simulink model "quietdriver"  (R2024b)
settings: Solver=FixedStepAuto  StartTime=0.0  StopTime=100  RelTol=1e-3
libraries: robotlib x5
settings Model: Creator=sprinkle  LastModifiedBy=fafac
settings OptimizationCC: DefaultParameterBehavior=Inlined  EnhancedBackFolding=on  PassReuseOutputArgsAs=Individual arguments  ZeroExternalMemoryAtStartup=off  ZeroInternalMemoryAtStartup=off  MaxStackSize=64  OptimizeBlockOrder=speed  DifferentSizesBufferReuse=on  OptimizationCustomize=off  EfficientTunableParamExpr=on
settings DebuggingCC: ParameterTunabilityLossMsg=error
settings HardwareCC: ProdBitPerPointer=32  ProdBitPerSizeT=32  ProdBitPerPtrDiffT=32  ProdLargestAtomicFloat=None  ProdIntDivRoundTo=Undefined  ProdEndianess=Unspecified  ProdWordSize=32  ProdHWDeviceType=Generic->Unspecified (assume 32-bit Generic)
settings SFSimCC: MATLABDynamicMemAlloc=off  SimTargetLang=C++
settings RTWCC: Description=Embedded Coder  SystemTargetFile=ert.tlc  HardwareBoard=Robot Operating System (ROS)  TLCOptions="-aInlineSetEventsForThisBaseRateFcn=TLC_FALSE -aSuppressMultiTaskScheduler=TLC_FALSE  -aRateBasedStepFcn=0"  TemplateMakefile=ert_default_tmf  Toolchain=Catkin  TargetLang=C++  GPUComputeCapability=3.5
settings CodeAppCC: ForceParamTrailComments=on  IgnoreCustomStorageClasses=off  OperatorAnnotations=on  SimulinkDataObjDesc=on  SFDataObjDesc=on  InsertBlockDesc=on
settings ERTTargetCC: CodeInterfacePackaging=C++ class  SupportContinuousTime=on  RootIOFormat=Structure reference

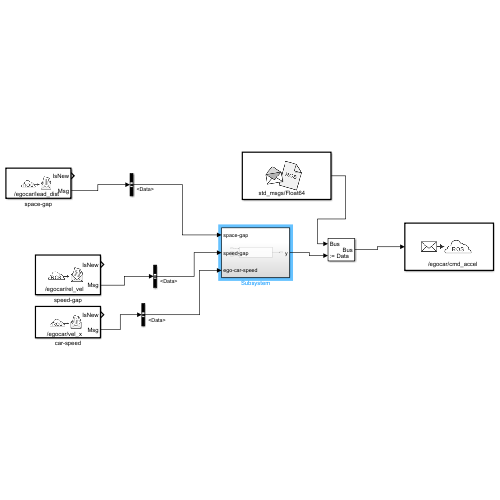
[thumbnail: Simulink's stored preview of the top-level diagram]
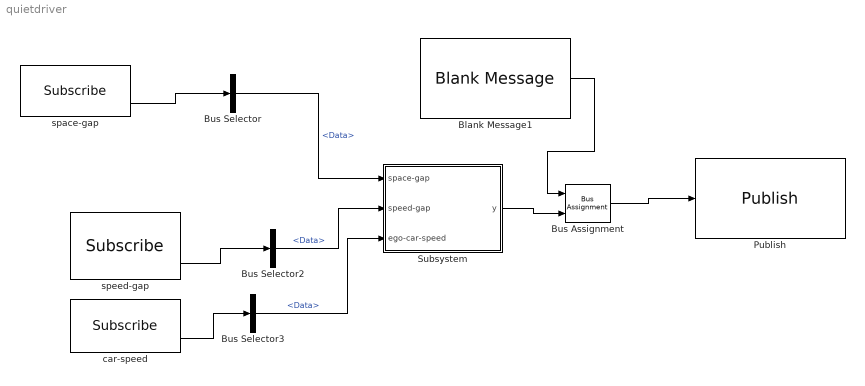
== system quietdriver ==
  Blank Message1 : robotlib/Blank Message  messageClass=Message  entityType=std_msgs/Float64  messageType=std_msgs/Float64  SampleTime=inf  legacyBusStruct=off
  Bus Assignment : BusAssignment  AssignedSignals=Data
  Bus Selector : BusSelector  OutputSignals=Data
  Bus Selector2 : BusSelector  OutputSignals=Data
  Bus Selector3 : BusSelector  OutputSignals=Data
  Publish : robotlib/Publish  topicSource=Specify your own  topic=/egocar/cmd_accel  messageType=std_msgs/Float64  legacyBusStruct=off  messageQueueLength=1
  Subsystem : Subsystem
  car-speed : robotlib/Subscribe  topicSource=Specify your own  topic=/egocar/vel_x  messageType=std_msgs/Float64  SampleTime=0.2  legacyBusStruct=off  messageQueueLength=1
  space-gap : robotlib/Subscribe  topicSource=Specify your own  topic=/egocar/lead_dist  messageType=std_msgs/Float64  SampleTime=0.2  legacyBusStruct=off  messageQueueLength=1
  speed-gap : robotlib/Subscribe  topicSource=Specify your own  topic=/egocar/rel_vel  messageType=std_msgs/Float64  SampleTime=0.2  legacyBusStruct=off  messageQueueLength=1
  wires:
  Subsystem/1(y) -> Bus Assignment/2
  Bus Assignment/1 -> Publish/1
  Blank Message1/1 -> Bus Assignment/1
  speed-gap/2 -> Bus Selector2/1
  Bus Selector2/1 -> Subsystem/2(speed-gap)  "<Data>"
  car-speed/2 -> Bus Selector3/1
  Bus Selector3/1 -> Subsystem/3(ego-car-speed)  "<Data>"
  space-gap/2 -> Bus Selector/1
  Bus Selector/1 -> Subsystem/1(space-gap)  "<Data>"

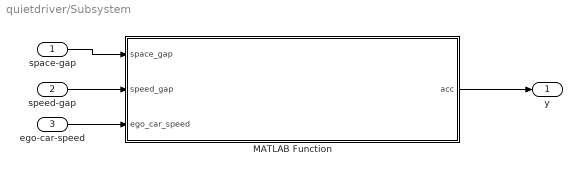
== system quietdriver/Subsystem ==
  space-gap : Inport
  speed-gap : Inport  Port=2
  ego-car-speed : Inport  Port=3
  MATLAB Function : MATLAB Function  TreatAsAtomicUnit=on
  y : Outport  OutDataTypeStr=double  LockScale=on
  wires:
  space-gap/1 -> MATLAB Function/1(space_gap)
  speed-gap/1 -> MATLAB Function/2(speed_gap)
  ego-car-speed/1 -> MATLAB Function/3(ego_car_speed)
  MATLAB Function/1(acc) -> y/1

== matlab function quietdriver/Subsystem/MATLAB Function ==
  data: space_gap input; acc output; speed_gap input; ego_car_speed input
function acc = fcn(space_gap, speed_gap, ego_car_speed)
    % Car Following Model implementation
    % Inputs:
    % space_gap: Distance to the leading vehicle [m]
    % speed_gap: Velocity difference with leading vehicle [m/s]
    % ego_car_speed: Current velocity of ego vehicle [m/s]
    % Output:
    % acc: Calculated acceleration [m/s^2]

    % Model parameters
    alpha = 0.05;     % Space gap sensitivity
    beta = 0.6;      % Speed gap sensitivity
    % gamma = 0.1;     % Acceleration gap sensitivity
    time_gap = 4;    % Desired time gap [s]
    
    % Calculate desired space gap
    desired_space = (ego_car_speed + 0.5) * time_gap;
    
    % Calculate space gap component (acc1)
    acc1 = alpha * (space_gap - desired_space);
    
    % Calculate speed component (acc2)
    acc2 = beta * speed_gap;
    
    % Calculate weight based on time gap difference
    % Weight is 1 if absolute difference between actual and desired time gap >= 1
    % Weight is 0 otherwise
    actual_time_gap = space_gap / (ego_car_speed + 0.5);
    weight = double(abs(actual_time_gap - time_gap) >= 1);
    
    % Combine accelerations using weight
    acc = acc1 + weight * acc2;
    % acc = acc1
    % % Add comfort acceleration term
    % comfort_term = gamma * (1 - (ego_car_speed/30)^2);  % Assuming 30 m/s as desired speed
    % acc = acc + comfort_term;
    
    % Clip acceleration within safe bounds
    acc = min(max(acc, -3), 1.5);
end
